simulink model "TrigSubsysFallschirm"  (R2018b)
settings: Solver=VariableStepAuto  StartTime=0.0  StopTime=inf  FixedStep=0.1  RelTol=1e-3  EnableMultiTasking=on
model workspace (MAT data in the model file):
  AFS = 30
  AS = 0.5
  DT = 3
  cw = 1.3
  g = 9.81
  h0 = 300
  h1 = 75
  m = 85
  rho = 1.2
  v0 = 0
settings Model: Creator=Reichl  LastModifiedBy=Reichl
settings DataIOCC: SaveFormat=Array
settings OptimizationCC: LifeSpan=inf
settings DebuggingCC: SolverPrmCheckMsg=warning  AllowSymbolicDim=off  SFUnexpectedBacktrackingDiag=warning  SFNoUnconditionalDefaultTransitionDiag=warning  SFExecutionAtInitializationDiag=none
settings HardwareCC: ProdBitPerPointer=32  ProdBitPerSizeT=32  ProdBitPerPtrDiffT=32  ProdLargestAtomicFloat=None  ProdIntDivRoundTo=Undefined  ProdEndianess=Unspecified  ProdWordSize=32  ProdHWDeviceType=32-bit Generic
settings ModelReferenceCC: PropagateSignalLabelsOutOfModel=off
settings SFSimCC: SimUseLocalCustomCode=off
settings RTWCC: RTWUseLocalCustomCode=off
settings CodeAppCC: StateflowObjectComments=on
settings GRTTargetCC: TargetLangStandard=C89/C90 (ANSI)  GeneratePreprocessorConditionals=Disable all
settings ConfigComp: CovMetricSettings=dw  CovHtmlReporting=on  CovSaveCumulativeToWorkspaceVar=on  CovSaveSingleToWorkspaceVar=on  CovExternalEMLEnable=off  CovSFcnEnable=off

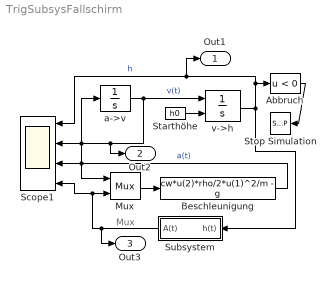
== system TrigSubsysFallschirm ==
  note: Mux
  Abbruch : Fcn  Expr=u < 0
  Beschleunigung : Fcn  Expr=cw*u(2)*rho/2*u(1)^2/m - g
  Mux : Mux  Inputs=2
      settings: DisplayOption=signals
  Scope1 : Scope  NumInputPorts=4
  Starthöhe : Constant  Value=h0
  Stop Simulation : Stop
  Subsystem : Subsystem
  a->v : Integrator  InitialCondition=v0
  v->h : Integrator  InitialConditionSource=external
  Out1 : Outport
  Out2 : Outport  Port=2
  Out3 : Outport  Port=3
  wires:
  a->v/1 -> v->h/1, Out2/1, Scope1/2, Mux/1  "v(t)"
  v->h/1 -> Out1/1, Scope1/1, Abbruch/1, Subsystem/1(h(t))  "h"
  Abbruch/1 -> Stop Simulation/1
  Starthöhe/1 -> v->h/2
  Mux/1 -> Beschleunigung/1
  Beschleunigung/1 -> a->v/1, Scope1/3  "a(t)"
  Subsystem/1(" A(t)") -> Out3/1, Scope1/4, Mux/2

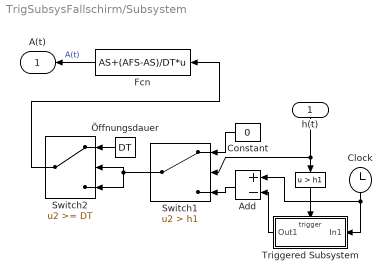
== system TrigSubsysFallschirm/Subsystem ==
  h(t) : Inport
  " " : Fcn  Expr=u > h1
  Add : Sum  Inputs=+-
  Clock : Clock
  Constant : Constant  Value=0
  Fcn : Fcn  Expr=AS+(AFS-AS)/DT*u
  Switch1 : Switch  Criteria=u2 > Threshold  Threshold=h1
  Switch2 : Switch  Threshold=DT
  Triggered Subsystem : Subsystem  TreatAsAtomicUnit=on
  Öffnungsdauer : Constant  Value=DT
  " A(t)" : Outport
  wires:
  h(t)/1 -> Switch1/2, " "/1
  Clock/1 -> Add/1, Triggered Subsystem/1(In1)
  Constant/1 -> Switch1/1
  " "/1 -> Triggered Subsystem/Trigger
  Triggered Subsystem/1(Out1) -> Add/2
  Add/1 -> Switch1/3
  Öffnungsdauer/1 -> Switch2/1
  Switch2/1 -> Fcn/1
  Switch1/1 -> Switch2/2, Switch2/3
  Fcn/1 -> " A(t)"/1  "A(t)"

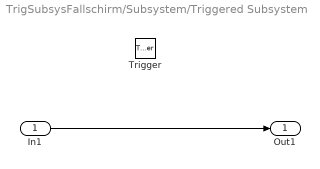
== system TrigSubsysFallschirm/Subsystem/Triggered Subsystem ==
  In1 : Inport
  Trigger : TriggerPort  TriggerType=falling  VariantControl=Variant
  Out1 : Outport
  wires:
  In1/1 -> Out1/1
